simulink model "ES250A_BattVltg"  (R2013b)
settings: Solver=ode45  StartTime=0.0  StopTime=Inf  RelTol=1e-3
values from neighbouring files (symbols this model uses):
  BattVltgCorrlnSysMinVltg = DataDict.ImprtdCal    [ES250A_BattVltg_DataDict.m]
  BattVltgSwdMax = DataDict.Calibration    [ES250A_BattVltg_DataDict.m]
  BRDGFLTVLTG_VOLT_F32 = DataDict.Constant    [ES250A_BattVltg_DataDict.m]
  BrdgVltgMax = DataDict.Calibration    [ES250A_BattVltg_DataDict.m]
settings Model: Creator=NZG49T  LastModifiedBy=nzg49t

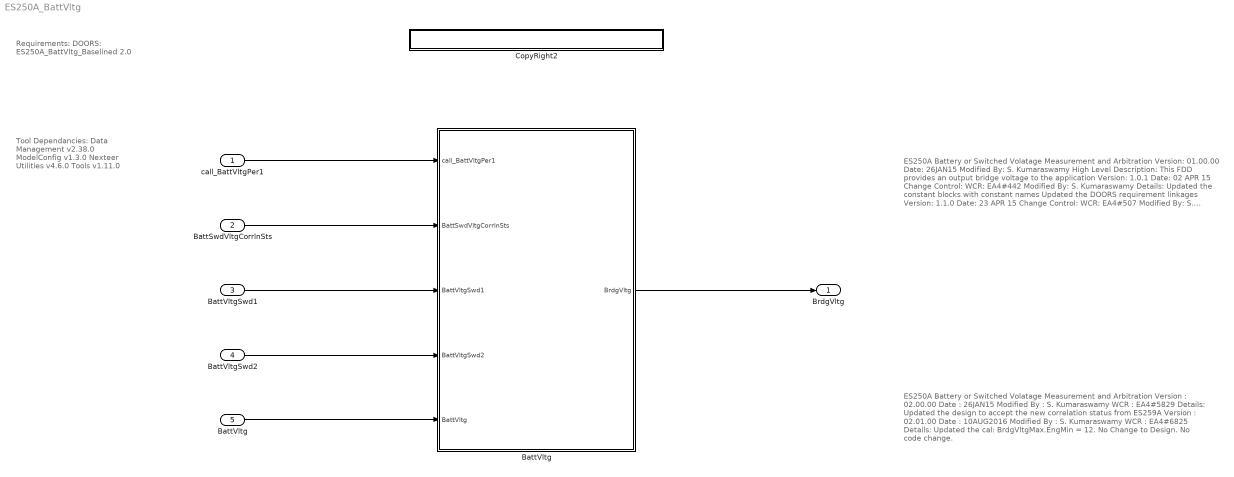
== system ES250A_BattVltg ==
  note: ES250A Battery or Switched Volatage Measurement and Arbitration
      |
      | Version: 01.00.00
      | Date: 26JAN15
      | Modified By: S. Kumaraswamy
      |
      | High Level Description:
      | This FDD provides an output bridge voltage to the application
      |
      | Version: 1.0.1
      | Date: 02 APR 15
      | Change Control: WCR: EA4#442
      | Modified By: S. Kumaraswamy
      | Details:
      | 	Updated the constant blocks with constant names
      | 	Updated the DOORS requirement linkages
      |
      | Version: 1.1.0
      | Date: 23 APR 15
      | Change Control: WCR: EA4#507
      | Modified By: S. Kumaraswamy
      | Details:
      | 	Updated the ES250A_BattVltg_DataDict.m file to change the range on inputs
  note: Tool Dependancies:
      |
      |    Data Management v2.38.0
      |    ModelConfig v1.3.0
      |    Nexteer Utilities v4.6.0
      |    Tools v1.11.0
  note: Requirements:
      |
      | DOORS: ES250A_BattVltg_Baselined 2.0
  note: ES250A Battery or Switched Volatage Measurement and Arbitration
      |
      | Version		: 02.00.00
      | Date		: 26JAN15
      | Modified By	: S. Kumaraswamy
      | WCR		: EA4#5829
      | Details:
      | 	Updated the design to accept the new correlation status from ES259A
      |
      | Version		: 02.01.00
      | Date		: 10AUG2016
      | Modified By	: S. Kumaraswamy
      | WCR		: EA4#6825
      | Details:
      | 	Updated the cal: BrdgVltgMax.EngMin = 12.
      | 	No Change to Design. No code change.
  call_BattVltgPer1 : Inport
  BattSwdVltgCorrlnSts : Inport  RequirementInfo={'linktype_rmi_doors' '000089be (/ESG Group/FDD Module Requirements/ES FDDs/ES-250A Battery and Switched Battery New Template)' '#ES250A_59' 'true' 'REQ:ES250A_59' '' } %GIDa_a11c860d_d132_4daf_a264_4400bd00e18c  Port=2
  BattVltgSwd1 : Inport  RequirementInfo={'linktype_rmi_doors' '000089be (/ESG Group/FDD Module Requirements/ES FDDs/ES-250A Battery and Switched Battery New Template)' '#ES250A_49' 'true' 'REQ:ES250A_49' '' } %GIDa_91354ed7_7d91_4356_a4ba_a513af450a0f  Port=3
  BattVltgSwd2 : Inport  RequirementInfo={'linktype_rmi_doors' '000089be (/ESG Group/FDD Module Requirements/ES FDDs/ES-250A Battery and Switched Battery New Template)' '#ES250A_60' 'true' 'REQ:ES250A_60' '' } %GIDa_49a2a00d_979f_48d9_9651_cd1224b822ec  Port=4
  "BattVltg " : Inport  RequirementInfo={'linktype_rmi_doors' '000089be (/ESG Group/FDD Module Requirements/ES FDDs/ES-250A Battery and Switched Battery New Template)' '#ES250A_48' 'true' 'REQ:ES250A_48' '' } %GIDa_3012d6f7_103b_47aa_89dd_d3628ff57ae0  Port=5
  BattVltg : Subsystem
  CopyRight2 : Subsystem  Description=|  mask(Copyright Information){none=on}
      | Copyright info block.                                               
      |                                                                     
      | Place copyright information at the top of every subsystem in design.
      mask prompts: none "No parameters"
      mask help: Place copyright information at the top of every subsystem in design.
      mask Display:
      | NxtrConf = 'Nexteer Confidential';
      | 
      | sys = bdroot; %handle for the current model ("system")
      | first = get_param(sys,'Created');
      | first = first(end-3:end);  %year is last four digits
      | 
      | last = get_param(sys,'LastModifiedDate');
      | if isempty(last)
      |     last = datestr(now,'yyyy');
      | else
      |     last = last(end-3:end);
      | end
      | 
      | if strcmp(first,last)
      |     fprintf('%s -- Copyright %s Nexteer',NxtrConf,first)
      | else
      |     fprintf('%s -- %s%s- %s Nexteer',NxtrConf,char(169),first,last)
      | end
  BrdgVltg : Outport  RequirementInfo={'linktype_rmi_doors' '000089be (/ESG Group/FDD Module Requirements/ES FDDs/ES-250A Battery and Switched Battery New Template)' '#ES250A_51' 'true' 'REQ:ES250A_51' '' } %GIDa_b80be137_a87b_4a79_92b7_89eced009269
  wires:
  BattVltg/1(BrdgVltg) -> BrdgVltg/1
  call_BattVltgPer1/1 -> BattVltg/1(call_BattVltgPer1)
  BattSwdVltgCorrlnSts/1 -> BattVltg/2(BattSwdVltgCorrlnSts)
  BattVltgSwd1/1 -> BattVltg/3(BattVltgSwd1)
  BattVltgSwd2/1 -> BattVltg/4(BattVltgSwd2)
  "BattVltg "/1 -> BattVltg/5(BattVltg)

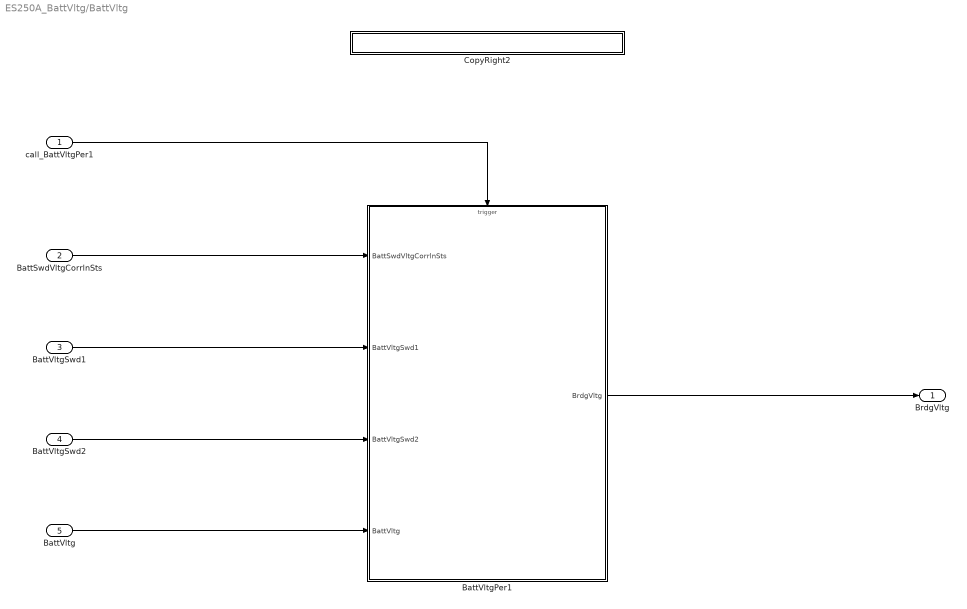
== system ES250A_BattVltg/BattVltg ==
  call_BattVltgPer1 : Inport
  BattSwdVltgCorrlnSts : Inport  RequirementInfo={'linktype_rmi_doors' '000089be (/ESG Group/FDD Module Requirements/ES FDDs/ES-250A Battery and Switched Battery New Template)' '#ES250A_59' 'true' 'REQ:ES250A_59' '' } %GIDa_e8385414_c5b7_4a96_916c_eabf55c4b14f  Port=2
  BattVltgSwd1 : Inport  RequirementInfo={'linktype_rmi_doors' '000089be (/ESG Group/FDD Module Requirements/ES FDDs/ES-250A Battery and Switched Battery New Template)' '#ES250A_49' 'true' 'REQ:ES250A_49' '' } %GIDa_5d2ad728_7230_4611_be80_0b164196a4c4  Port=3
  BattVltgSwd2 : Inport  RequirementInfo={'linktype_rmi_doors' '000089be (/ESG Group/FDD Module Requirements/ES FDDs/ES-250A Battery and Switched Battery New Template)' '#ES250A_60' 'true' 'REQ:ES250A_60' '' } %GIDa_aca025b3_6872_471e_9ce2_4632c3bd27ab  Port=4
  BattVltg : Inport  RequirementInfo={'linktype_rmi_doors' '000089be (/ESG Group/FDD Module Requirements/ES FDDs/ES-250A Battery and Switched Battery New Template)' '#ES250A_48' 'true' 'REQ:ES250A_48' '' } %GIDa_446049f3_a572_45b9_9ea0_5a0b2ee9b9f3  Port=5
  BattVltgPer1 : Subsystem
  CopyRight2 : Subsystem  Description=|  mask(Copyright Information){none=on}
      | Copyright info block.                                               
      |                                                                     
      | Place copyright information at the top of every subsystem in design.
      mask prompts: none "No parameters"
      mask help: Place copyright information at the top of every subsystem in design.
      mask Display:
      | NxtrConf = 'Nexteer Confidential';
      | 
      | sys = bdroot; %handle for the current model ("system")
      | first = get_param(sys,'Created');
      | first = first(end-3:end);  %year is last four digits
      | 
      | last = get_param(sys,'LastModifiedDate');
      | if isempty(last)
      |     last = datestr(now,'yyyy');
      | else
      |     last = last(end-3:end);
      | end
      | 
      | if strcmp(first,last)
      |     fprintf('%s -- Copyright %s Nexteer',NxtrConf,first)
      | else
      |     fprintf('%s -- %s%s- %s Nexteer',NxtrConf,char(169),first,last)
      | end
  BrdgVltg : Outport  RequirementInfo={'linktype_rmi_doors' '000089be (/ESG Group/FDD Module Requirements/ES FDDs/ES-250A Battery and Switched Battery New Template)' '#ES250A_51' 'true' 'REQ:ES250A_51' '' } %GIDa_1df96ea3_bed0_4e73_9e35_964b8173dbf2
  wires:
  call_BattVltgPer1/1 -> BattVltgPer1/Trigger
  BattVltgSwd2/1 -> BattVltgPer1/3(BattVltgSwd2)
  BattVltgSwd1/1 -> BattVltgPer1/2(BattVltgSwd1)
  BattSwdVltgCorrlnSts/1 -> BattVltgPer1/1(BattSwdVltgCorrlnSts)
  BattVltg/1 -> BattVltgPer1/4(BattVltg)
  BattVltgPer1/1(BrdgVltg) -> BrdgVltg/1

== system ES250A_BattVltg/CopyRight2 ==

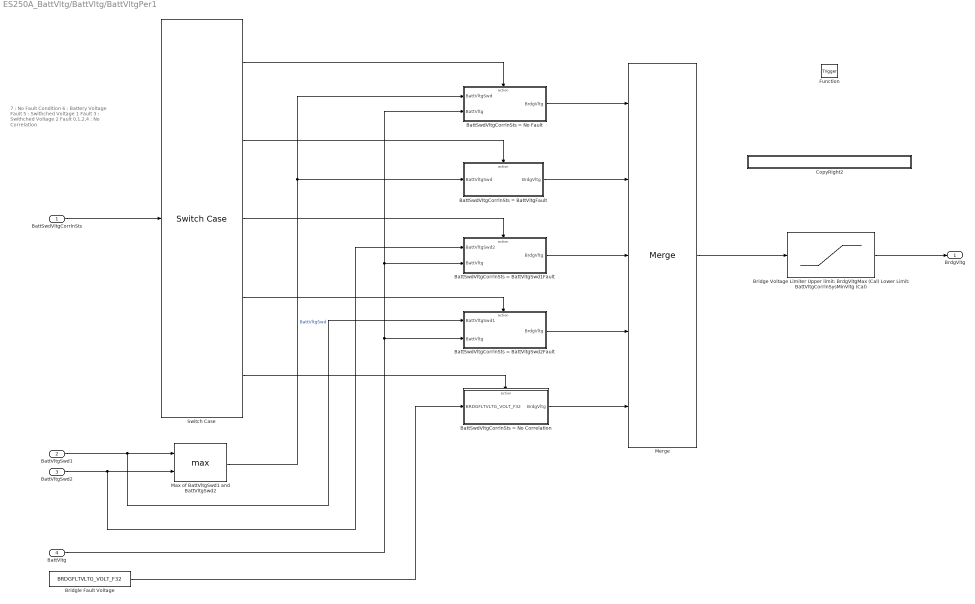
== system ES250A_BattVltg/BattVltg/BattVltgPer1 ==
  note: 7		: No Fault Condition
      | 6		: Battery Voltage Fault
      | 5		: Swithched Voltage 1 Fault
      | 3		: Swithched Voltage 2 Fault
      | 0,1,2,4	: No Correlation
  BattSwdVltgCorrlnSts : Inport
  BattVltgSwd1 : Inport  Port=2
  BattVltgSwd2 : Inport  Port=3
  BattVltg : Inport  Port=4
  Function : TriggerPort  TriggerType=function-call
  BattSwdVltgCorrlnSts = BattVltgFault : Subsystem  RequirementInfo={'linktype_rmi_doors' '000089be (/ESG Group/FDD Module Requirements/ES FDDs/ES-250A Battery and Switched Battery New Template)' '#ES250A_70' 'true' 'REQ:ES250A_70' '' } %GIDa_1e80a747_e46b_4fae_a462_c14971ea2063  TreatAsAtomicUnit=on
  BattSwdVltgCorrlnSts = BattVltgSwd1Fault : Subsystem  RequirementInfo={'linktype_rmi_doors' '000089be (/E-STEER Core/SubSystem Specifications/Electrical Actuator/Control Module/FDD Module Requirements/EA4/ES250A_BattVltg)' '#ES250A_71' 'true' 'REQ:ES250A_71' '' ; 'linktype_rmi_doors' '000089be (/E-STEER Core/SubSystem Specifications/Electrical Actuator/Control Module/FDD Module Requirements/EA4/ES250A_BattVltg)' '#ES250A_74' 'true' 'REQ:ES250A_74' '' } %GIDa_d2edab66_9a38_4fa0_805c_5347de679304  TreatAsAtomicUnit=on
  BattSwdVltgCorrlnSts = BattVltgSwd2Fault : Subsystem  RequirementInfo={'linktype_rmi_doors' '000089be (/E-STEER Core/SubSystem Specifications/Electrical Actuator/Control Module/FDD Module Requirements/EA4/ES250A_BattVltg)' '#ES250A_71' 'true' 'REQ:ES250A_71' '' ; 'linktype_rmi_doors' '000089be (/E-STEER Core/SubSystem Specifications/Electrical Actuator/Control Module/FDD Module Requirements/EA4/ES250A_BattVltg)' '#ES250A_73' 'true' 'REQ:ES250A_73' '' } %GIDa_b90dafad_55ba_4f29_80ae_7ffeed94569b  TreatAsAtomicUnit=on
  BattSwdVltgCorrlnSts = No Correlation : Subsystem  RequirementInfo={'linktype_rmi_doors' '000089be (/E-STEER Core/SubSystem Specifications/Electrical Actuator/Control Module/FDD Module Requirements/EA4/ES250A_BattVltg)' '#ES250A_69' 'true' 'REQ:ES250A_69' '' } %GIDa_00f660ee_d345_4718_bc3f_0f212dfcf13e  TreatAsAtomicUnit=on
  BattSwdVltgCorrlnSts = No Fault : Subsystem  RequirementInfo={'linktype_rmi_doors' '000089be (/E-STEER Core/SubSystem Specifications/Electrical Actuator/Control Module/FDD Module Requirements/EA4/ES250A_BattVltg)' '#ES250A_71' 'true' 'REQ:ES250A_71' '' ; 'linktype_rmi_doors' '000089be (/E-STEER Core/SubSystem Specifications/Electrical Actuator/Control Module/FDD Module Requirements/EA4/ES250A_BattVltg)' '#ES250A_72' 'true' 'REQ:ES250A_72' '' } %GIDa_5403e315_0859_46da_b9ef_39481c3f6656  TreatAsAtomicUnit=on
  Bridge Voltage Limiter Upper limit: BrdgVltgMax (Cal) Lower Limit: BattVltgCorrlnSysMinVltg (Cal) : Saturate  RequirementInfo={'linktype_rmi_doors' '000089be (/ESG Group/FDD Module Requirements/ES FDDs/ES-250A Battery and Switched Battery New Template)' '#ES250A_77' 'true' 'REQ:ES250A_77' '' } %GIDa_140e9a93_79da_47f9_8f89_a5c416ccae8e  UpperLimit=BrdgVltgMax  LowerLimit=BattVltgCorrlnSysMinVltg
  Bridgle Fault Voltage : Constant  Value=BRDGFLTVLTG_VOLT_F32  OutDataTypeStr=single
  CopyRight2 : Subsystem  Description=|  mask(Copyright Information){none=on}
      | Copyright info block.                                               
      |                                                                     
      | Place copyright information at the top of every subsystem in design.
      mask prompts: none "No parameters"
      mask help: Place copyright information at the top of every subsystem in design.
      mask Display:
      | NxtrConf = 'Nexteer Confidential';
      | 
      | sys = bdroot; %handle for the current model ("system")
      | first = get_param(sys,'Created');
      | first = first(end-3:end);  %year is last four digits
      | 
      | last = get_param(sys,'LastModifiedDate');
      | if isempty(last)
      |     last = datestr(now,'yyyy');
      | else
      |     last = last(end-3:end);
      | end
      | 
      | if strcmp(first,last)
      |     fprintf('%s -- Copyright %s Nexteer',NxtrConf,first)
      | else
      |     fprintf('%s -- %s%s- %s Nexteer',NxtrConf,char(169),first,last)
      | end
  Max of BattVltgSwd1 and BattVltgSwd2 : MinMax  Function=max  Inputs=2  ZeroCross=off
  Merge : Merge  Inputs=5
  Switch Case : SwitchCase  CaseConditions={7,6,5,3}
  BrdgVltg : Outport
  wires:
  BattSwdVltgCorrlnSts/1 -> Switch Case/1
  BattVltgSwd1/1 -> BattSwdVltgCorrlnSts = BattVltgSwd2Fault/1(BattVltgSwd1), Max of BattVltgSwd1 and BattVltgSwd2/1
  Max of BattVltgSwd1 and BattVltgSwd2/1 -> BattSwdVltgCorrlnSts = No Fault/1(BattVltgSwd), BattSwdVltgCorrlnSts = BattVltgFault/1(BattVltgSwd)  "BattVltgSwd"
  Switch Case/5 -> BattSwdVltgCorrlnSts = No Correlation/Action
  BattVltgSwd2/1 -> Max of BattVltgSwd1 and BattVltgSwd2/2, BattSwdVltgCorrlnSts = BattVltgSwd1Fault/1(BattVltgSwd2)
  BattSwdVltgCorrlnSts = No Correlation/1(BrdgVltg) -> Merge/5
  Bridgle Fault Voltage/1 -> BattSwdVltgCorrlnSts = No Correlation/1(BRDGFLTVLTG_VOLT_F32)
  BattVltg/1 -> BattSwdVltgCorrlnSts = No Fault/2(BattVltg), BattSwdVltgCorrlnSts = BattVltgSwd1Fault/2(BattVltg), BattSwdVltgCorrlnSts = BattVltgSwd2Fault/2(BattVltg)
  BattSwdVltgCorrlnSts = No Fault/1(BrdgVltg) -> Merge/1
  Switch Case/1 -> BattSwdVltgCorrlnSts = No Fault/Action
  Merge/1 -> Bridge Voltage Limiter Upper limit: BrdgVltgMax (Cal) Lower Limit: BattVltgCorrlnSysMinVltg (Cal)/1
  Bridge Voltage Limiter Upper limit: BrdgVltgMax (Cal) Lower Limit: BattVltgCorrlnSysMinVltg (Cal)/1 -> BrdgVltg/1
  Switch Case/2 -> BattSwdVltgCorrlnSts = BattVltgFault/Action
  Switch Case/3 -> BattSwdVltgCorrlnSts = BattVltgSwd1Fault/Action
  Switch Case/4 -> BattSwdVltgCorrlnSts = BattVltgSwd2Fault/Action
  BattSwdVltgCorrlnSts = BattVltgFault/1(BrdgVltg) -> Merge/2
  BattSwdVltgCorrlnSts = BattVltgSwd1Fault/1(BrdgVltg) -> Merge/3
  BattSwdVltgCorrlnSts = BattVltgSwd2Fault/1(BrdgVltg) -> Merge/4

== system ES250A_BattVltg/BattVltg/CopyRight2 ==

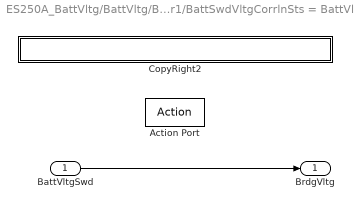
== system ES250A_BattVltg/BattVltg/BattVltgPer1/BattSwdVltgCorrlnSts = BattVltgFault ==
  BattVltgSwd : Inport
  Action Port : ActionPort  ActionType=case
  CopyRight2 : Subsystem  Description=|  mask(Copyright Information){none=on}
      | Copyright info block.                                               
      |                                                                     
      | Place copyright information at the top of every subsystem in design.
      mask prompts: none "No parameters"
      mask help: Place copyright information at the top of every subsystem in design.
      mask Display:
      | NxtrConf = 'Nexteer Confidential';
      | 
      | sys = bdroot; %handle for the current model ("system")
      | first = get_param(sys,'Created');
      | first = first(end-3:end);  %year is last four digits
      | 
      | last = get_param(sys,'LastModifiedDate');
      | if isempty(last)
      |     last = datestr(now,'yyyy');
      | else
      |     last = last(end-3:end);
      | end
      | 
      | if strcmp(first,last)
      |     fprintf('%s -- Copyright %s Nexteer',NxtrConf,first)
      | else
      |     fprintf('%s -- %s%s- %s Nexteer',NxtrConf,char(169),first,last)
      | end
  BrdgVltg : Outport
  wires:
  BattVltgSwd/1 -> BrdgVltg/1

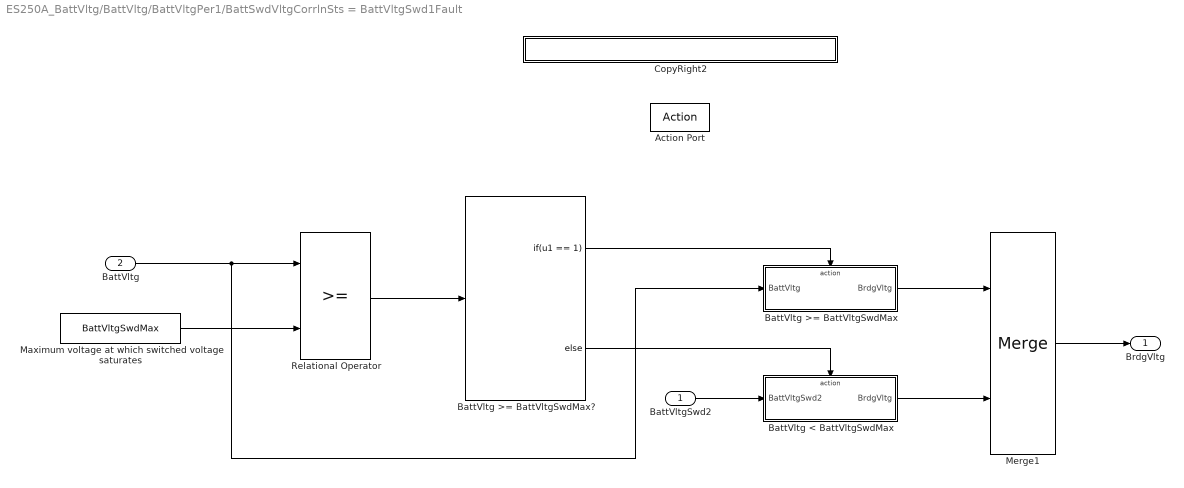
== system ES250A_BattVltg/BattVltg/BattVltgPer1/BattSwdVltgCorrlnSts = BattVltgSwd1Fault ==
  BattVltgSwd2 : Inport
  BattVltg : Inport  Port=2
  Action Port : ActionPort  ActionType=case
  BattVltg < BattVltgSwdMax : Subsystem  RequirementInfo={'linktype_rmi_doors' '000089be (/ESG Group/FDD Module Requirements/ES FDDs/ES-250A Battery and Switched Battery New Template)' '#ES250A_74' 'true' 'REQ:ES250A_74' '' } %GIDa_07292b91_eb89_4c3a_b17b_a04f2de4c9d3  TreatAsAtomicUnit=on
  BattVltg >= BattVltgSwdMax : Subsystem  RequirementInfo={'linktype_rmi_doors' '000089be (/ESG Group/FDD Module Requirements/ES FDDs/ES-250A Battery and Switched Battery New Template)' '#ES250A_71' 'true' 'REQ:ES250A_71' '' } %GIDa_bcfe97d8_f970_4b6a_b766_e1f79e97ff7b  TreatAsAtomicUnit=on
  BattVltg >= BattVltgSwdMax? : If  IfExpression=u1 == 1
  CopyRight2 : Subsystem  Description=|  mask(Copyright Information){none=on}
      | Copyright info block.                                               
      |                                                                     
      | Place copyright information at the top of every subsystem in design.
      mask prompts: none "No parameters"
      mask help: Place copyright information at the top of every subsystem in design.
      mask Display:
      | NxtrConf = 'Nexteer Confidential';
      | 
      | sys = bdroot; %handle for the current model ("system")
      | first = get_param(sys,'Created');
      | first = first(end-3:end);  %year is last four digits
      | 
      | last = get_param(sys,'LastModifiedDate');
      | if isempty(last)
      |     last = datestr(now,'yyyy');
      | else
      |     last = last(end-3:end);
      | end
      | 
      | if strcmp(first,last)
      |     fprintf('%s -- Copyright %s Nexteer',NxtrConf,first)
      | else
      |     fprintf('%s -- %s%s- %s Nexteer',NxtrConf,char(169),first,last)
      | end
  Maximum voltage at which switched voltage saturates : Constant  Value=BattVltgSwdMax  OutDataTypeStr=single
  Merge1 : Merge
  Relational Operator : RelationalOperator  OutDataTypeStr=boolean
  BrdgVltg : Outport
  wires:
  BattVltg >= BattVltgSwdMax?/1 -> BattVltg >= BattVltgSwdMax/Action
  BattVltg >= BattVltgSwdMax?/2 -> BattVltg < BattVltgSwdMax/Action
  BattVltgSwd2/1 -> BattVltg < BattVltgSwdMax/1(BattVltgSwd2)
  BattVltg >= BattVltgSwdMax/1(BrdgVltg) -> Merge1/1
  BattVltg < BattVltgSwdMax/1(BrdgVltg) -> Merge1/2
  Merge1/1 -> BrdgVltg/1
  BattVltg/1 -> BattVltg >= BattVltgSwdMax/1(BattVltg), Relational Operator/1
  Maximum voltage at which switched voltage saturates/1 -> Relational Operator/2
  Relational Operator/1 -> BattVltg >= BattVltgSwdMax?/1

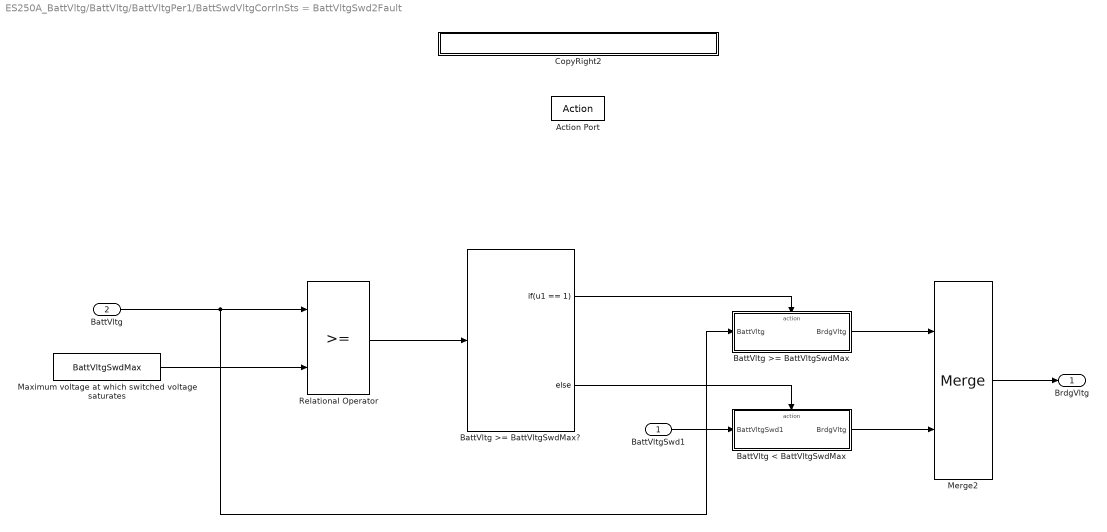
== system ES250A_BattVltg/BattVltg/BattVltgPer1/BattSwdVltgCorrlnSts = BattVltgSwd2Fault ==
  BattVltgSwd1 : Inport
  BattVltg : Inport  Port=2
  Action Port : ActionPort  ActionType=case
  BattVltg < BattVltgSwdMax : Subsystem  RequirementInfo={'linktype_rmi_doors' '000089be (/ESG Group/FDD Module Requirements/ES FDDs/ES-250A Battery and Switched Battery New Template)' '#ES250A_73' 'true' 'REQ:ES250A_73' '' } %GIDa_307ba01f_b79a_432e_bfbc_716903f8ff55  TreatAsAtomicUnit=on
  BattVltg >= BattVltgSwdMax : Subsystem  RequirementInfo={'linktype_rmi_doors' '000089be (/ESG Group/FDD Module Requirements/ES FDDs/ES-250A Battery and Switched Battery New Template)' '#ES250A_71' 'true' 'REQ:ES250A_71' '' } %GIDa_ba8018fa_2f9e_46d8_a7b7_d203f8c6e12a  TreatAsAtomicUnit=on
  BattVltg >= BattVltgSwdMax? : If  IfExpression=u1 == 1
  CopyRight2 : Subsystem  Description=|  mask(Copyright Information){none=on}
      | Copyright info block.                                               
      |                                                                     
      | Place copyright information at the top of every subsystem in design.
      mask prompts: none "No parameters"
      mask help: Place copyright information at the top of every subsystem in design.
      mask Display:
      | NxtrConf = 'Nexteer Confidential';
      | 
      | sys = bdroot; %handle for the current model ("system")
      | first = get_param(sys,'Created');
      | first = first(end-3:end);  %year is last four digits
      | 
      | last = get_param(sys,'LastModifiedDate');
      | if isempty(last)
      |     last = datestr(now,'yyyy');
      | else
      |     last = last(end-3:end);
      | end
      | 
      | if strcmp(first,last)
      |     fprintf('%s -- Copyright %s Nexteer',NxtrConf,first)
      | else
      |     fprintf('%s -- %s%s- %s Nexteer',NxtrConf,char(169),first,last)
      | end
  Maximum voltage at which switched voltage saturates : Constant  Value=BattVltgSwdMax  OutDataTypeStr=single
  Merge2 : Merge
  Relational Operator : RelationalOperator  OutDataTypeStr=boolean
  BrdgVltg : Outport
  wires:
  BattVltg/1 -> BattVltg >= BattVltgSwdMax/1(BattVltg), Relational Operator/1
  BattVltg >= BattVltgSwdMax?/1 -> BattVltg >= BattVltgSwdMax/Action
  BattVltg >= BattVltgSwdMax?/2 -> BattVltg < BattVltgSwdMax/Action
  BattVltgSwd1/1 -> BattVltg < BattVltgSwdMax/1(BattVltgSwd1)
  BattVltg >= BattVltgSwdMax/1(BrdgVltg) -> Merge2/1
  BattVltg < BattVltgSwdMax/1(BrdgVltg) -> Merge2/2
  Merge2/1 -> BrdgVltg/1
  Maximum voltage at which switched voltage saturates/1 -> Relational Operator/2
  Relational Operator/1 -> BattVltg >= BattVltgSwdMax?/1

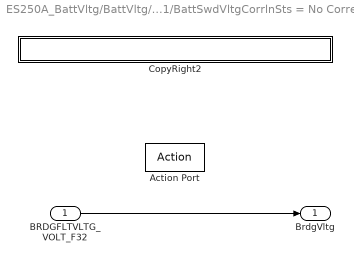
== system ES250A_BattVltg/BattVltg/BattVltgPer1/BattSwdVltgCorrlnSts = No Correlation ==
  BRDGFLTVLTG_VOLT_F32 : Inport
  Action Port : ActionPort  ActionType=default
  CopyRight2 : Subsystem  Description=|  mask(Copyright Information){none=on}
      | Copyright info block.                                               
      |                                                                     
      | Place copyright information at the top of every subsystem in design.
      mask prompts: none "No parameters"
      mask help: Place copyright information at the top of every subsystem in design.
      mask Display:
      | NxtrConf = 'Nexteer Confidential';
      | 
      | sys = bdroot; %handle for the current model ("system")
      | first = get_param(sys,'Created');
      | first = first(end-3:end);  %year is last four digits
      | 
      | last = get_param(sys,'LastModifiedDate');
      | if isempty(last)
      |     last = datestr(now,'yyyy');
      | else
      |     last = last(end-3:end);
      | end
      | 
      | if strcmp(first,last)
      |     fprintf('%s -- Copyright %s Nexteer',NxtrConf,first)
      | else
      |     fprintf('%s -- %s%s- %s Nexteer',NxtrConf,char(169),first,last)
      | end
  BrdgVltg : Outport
  wires:
  BRDGFLTVLTG_VOLT_F32/1 -> BrdgVltg/1

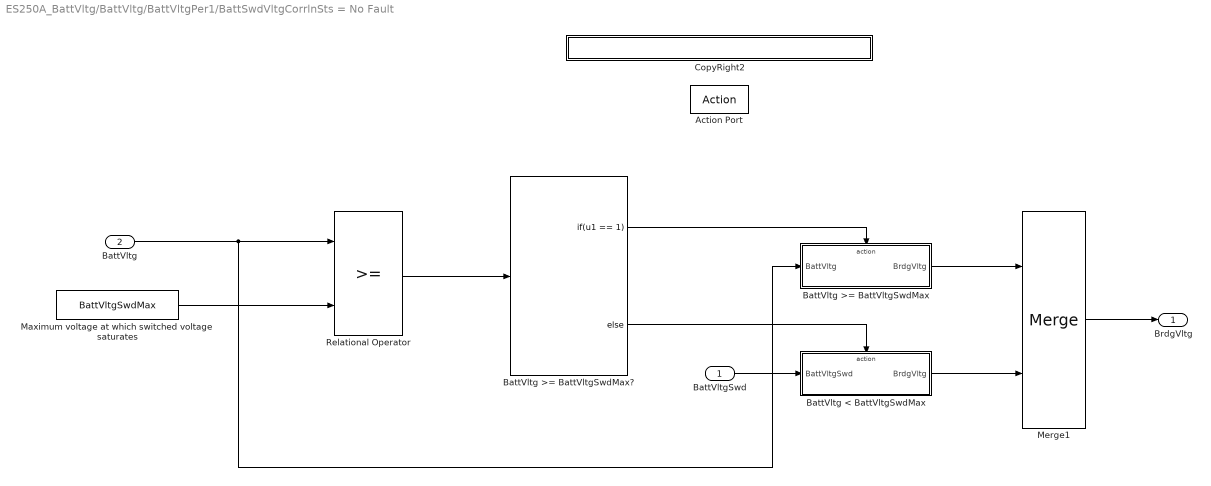
== system ES250A_BattVltg/BattVltg/BattVltgPer1/BattSwdVltgCorrlnSts = No Fault ==
  BattVltgSwd : Inport
  BattVltg : Inport  Port=2
  Action Port : ActionPort  ActionType=case
  BattVltg < BattVltgSwdMax : Subsystem  RequirementInfo={'linktype_rmi_doors' '000089be (/ESG Group/FDD Module Requirements/ES FDDs/ES-250A Battery and Switched Battery New Template)' '#ES250A_72' 'true' 'REQ:ES250A_72' '' } %GIDa_fc36a75c_2fdb_43c4_a531_122c5df0c909  TreatAsAtomicUnit=on
  BattVltg >= BattVltgSwdMax : Subsystem  RequirementInfo={'linktype_rmi_doors' '000089be (/ESG Group/FDD Module Requirements/ES FDDs/ES-250A Battery and Switched Battery New Template)' '#ES250A_71' 'true' 'REQ:ES250A_71' '' } %GIDa_4f6ba4fb_a439_4a78_8be4_0d81f695ed1e  TreatAsAtomicUnit=on
  BattVltg >= BattVltgSwdMax? : If  IfExpression=u1 == 1
  CopyRight2 : Subsystem  Description=|  mask(Copyright Information){none=on}
      | Copyright info block.                                               
      |                                                                     
      | Place copyright information at the top of every subsystem in design.
      mask prompts: none "No parameters"
      mask help: Place copyright information at the top of every subsystem in design.
      mask Display:
      | NxtrConf = 'Nexteer Confidential';
      | 
      | sys = bdroot; %handle for the current model ("system")
      | first = get_param(sys,'Created');
      | first = first(end-3:end);  %year is last four digits
      | 
      | last = get_param(sys,'LastModifiedDate');
      | if isempty(last)
      |     last = datestr(now,'yyyy');
      | else
      |     last = last(end-3:end);
      | end
      | 
      | if strcmp(first,last)
      |     fprintf('%s -- Copyright %s Nexteer',NxtrConf,first)
      | else
      |     fprintf('%s -- %s%s- %s Nexteer',NxtrConf,char(169),first,last)
      | end
  Maximum voltage at which switched voltage saturates : Constant  Value=BattVltgSwdMax  OutDataTypeStr=single
  Merge1 : Merge
  Relational Operator : RelationalOperator  OutDataTypeStr=boolean
  BrdgVltg : Outport
  wires:
  BattVltg/1 -> BattVltg >= BattVltgSwdMax/1(BattVltg), Relational Operator/1
  BattVltg >= BattVltgSwdMax?/1 -> BattVltg >= BattVltgSwdMax/Action
  BattVltg >= BattVltgSwdMax?/2 -> BattVltg < BattVltgSwdMax/Action
  BattVltgSwd/1 -> BattVltg < BattVltgSwdMax/1(BattVltgSwd)
  BattVltg >= BattVltgSwdMax/1(BrdgVltg) -> Merge1/1
  BattVltg < BattVltgSwdMax/1(BrdgVltg) -> Merge1/2
  Merge1/1 -> BrdgVltg/1
  Maximum voltage at which switched voltage saturates/1 -> Relational Operator/2
  Relational Operator/1 -> BattVltg >= BattVltgSwdMax?/1

== system ES250A_BattVltg/BattVltg/BattVltgPer1/CopyRight2 ==

== system ES250A_BattVltg/BattVltg/BattVltgPer1/BattSwdVltgCorrlnSts = BattVltgFault/CopyRight2 ==

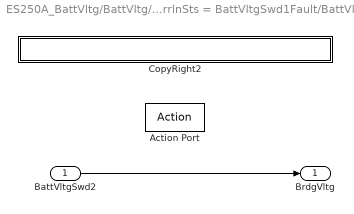
== system ES250A_BattVltg/BattVltg/BattVltgPer1/BattSwdVltgCorrlnSts = BattVltgSwd1Fault/BattVltg < BattVltgSwdMax ==
  BattVltgSwd2 : Inport
  Action Port : ActionPort  ActionType=else
  CopyRight2 : Subsystem  Description=|  mask(Copyright Information){none=on}
      | Copyright info block.                                               
      |                                                                     
      | Place copyright information at the top of every subsystem in design.
      mask prompts: none "No parameters"
      mask help: Place copyright information at the top of every subsystem in design.
      mask Display:
      | NxtrConf = 'Nexteer Confidential';
      | 
      | sys = bdroot; %handle for the current model ("system")
      | first = get_param(sys,'Created');
      | first = first(end-3:end);  %year is last four digits
      | 
      | last = get_param(sys,'LastModifiedDate');
      | if isempty(last)
      |     last = datestr(now,'yyyy');
      | else
      |     last = last(end-3:end);
      | end
      | 
      | if strcmp(first,last)
      |     fprintf('%s -- Copyright %s Nexteer',NxtrConf,first)
      | else
      |     fprintf('%s -- %s%s- %s Nexteer',NxtrConf,char(169),first,last)
      | end
  BrdgVltg : Outport
  wires:
  BattVltgSwd2/1 -> BrdgVltg/1

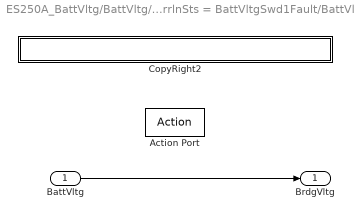
== system ES250A_BattVltg/BattVltg/BattVltgPer1/BattSwdVltgCorrlnSts = BattVltgSwd1Fault/BattVltg >= BattVltgSwdMax ==
  BattVltg : Inport
  Action Port : ActionPort  ActionType=then
  CopyRight2 : Subsystem  Description=|  mask(Copyright Information){none=on}
      | Copyright info block.                                               
      |                                                                     
      | Place copyright information at the top of every subsystem in design.
      mask prompts: none "No parameters"
      mask help: Place copyright information at the top of every subsystem in design.
      mask Display:
      | NxtrConf = 'Nexteer Confidential';
      | 
      | sys = bdroot; %handle for the current model ("system")
      | first = get_param(sys,'Created');
      | first = first(end-3:end);  %year is last four digits
      | 
      | last = get_param(sys,'LastModifiedDate');
      | if isempty(last)
      |     last = datestr(now,'yyyy');
      | else
      |     last = last(end-3:end);
      | end
      | 
      | if strcmp(first,last)
      |     fprintf('%s -- Copyright %s Nexteer',NxtrConf,first)
      | else
      |     fprintf('%s -- %s%s- %s Nexteer',NxtrConf,char(169),first,last)
      | end
  BrdgVltg : Outport
  wires:
  BattVltg/1 -> BrdgVltg/1

== system ES250A_BattVltg/BattVltg/BattVltgPer1/BattSwdVltgCorrlnSts = BattVltgSwd1Fault/CopyRight2 ==

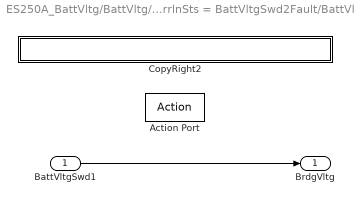
== system ES250A_BattVltg/BattVltg/BattVltgPer1/BattSwdVltgCorrlnSts = BattVltgSwd2Fault/BattVltg < BattVltgSwdMax ==
  BattVltgSwd1 : Inport
  Action Port : ActionPort  ActionType=else
  CopyRight2 : Subsystem  Description=|  mask(Copyright Information){none=on}
      | Copyright info block.                                               
      |                                                                     
      | Place copyright information at the top of every subsystem in design.
      mask prompts: none "No parameters"
      mask help: Place copyright information at the top of every subsystem in design.
      mask Display:
      | NxtrConf = 'Nexteer Confidential';
      | 
      | sys = bdroot; %handle for the current model ("system")
      | first = get_param(sys,'Created');
      | first = first(end-3:end);  %year is last four digits
      | 
      | last = get_param(sys,'LastModifiedDate');
      | if isempty(last)
      |     last = datestr(now,'yyyy');
      | else
      |     last = last(end-3:end);
      | end
      | 
      | if strcmp(first,last)
      |     fprintf('%s -- Copyright %s Nexteer',NxtrConf,first)
      | else
      |     fprintf('%s -- %s%s- %s Nexteer',NxtrConf,char(169),first,last)
      | end
  BrdgVltg : Outport
  wires:
  BattVltgSwd1/1 -> BrdgVltg/1

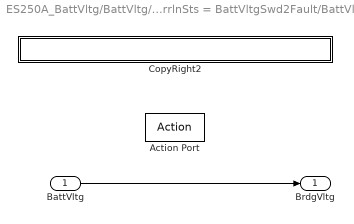
== system ES250A_BattVltg/BattVltg/BattVltgPer1/BattSwdVltgCorrlnSts = BattVltgSwd2Fault/BattVltg >= BattVltgSwdMax ==
  BattVltg : Inport
  Action Port : ActionPort  ActionType=then
  CopyRight2 : Subsystem  Description=|  mask(Copyright Information){none=on}
      | Copyright info block.                                               
      |                                                                     
      | Place copyright information at the top of every subsystem in design.
      mask prompts: none "No parameters"
      mask help: Place copyright information at the top of every subsystem in design.
      mask Display:
      | NxtrConf = 'Nexteer Confidential';
      | 
      | sys = bdroot; %handle for the current model ("system")
      | first = get_param(sys,'Created');
      | first = first(end-3:end);  %year is last four digits
      | 
      | last = get_param(sys,'LastModifiedDate');
      | if isempty(last)
      |     last = datestr(now,'yyyy');
      | else
      |     last = last(end-3:end);
      | end
      | 
      | if strcmp(first,last)
      |     fprintf('%s -- Copyright %s Nexteer',NxtrConf,first)
      | else
      |     fprintf('%s -- %s%s- %s Nexteer',NxtrConf,char(169),first,last)
      | end
  BrdgVltg : Outport
  wires:
  BattVltg/1 -> BrdgVltg/1

== system ES250A_BattVltg/BattVltg/BattVltgPer1/BattSwdVltgCorrlnSts = BattVltgSwd2Fault/CopyRight2 ==

== system ES250A_BattVltg/BattVltg/BattVltgPer1/BattSwdVltgCorrlnSts = No Correlation/CopyRight2 ==

== system ES250A_BattVltg/BattVltg/BattVltgPer1/BattSwdVltgCorrlnSts = No Fault/BattVltg < BattVltgSwdMax ==
  BattVltgSwd : Inport
  Action Port : ActionPort  ActionType=else
  CopyRight2 : Subsystem  Description=|  mask(Copyright Information){none=on}
      | Copyright info block.                                               
      |                                                                     
      | Place copyright information at the top of every subsystem in design.
      mask prompts: none "No parameters"
      mask help: Place copyright information at the top of every subsystem in design.
      mask Display:
      | NxtrConf = 'Nexteer Confidential';
      | 
      | sys = bdroot; %handle for the current model ("system")
      | first = get_param(sys,'Created');
      | first = first(end-3:end);  %year is last four digits
      | 
      | last = get_param(sys,'LastModifiedDate');
      | if isempty(last)
      |     last = datestr(now,'yyyy');
      | else
      |     last = last(end-3:end);
      | end
      | 
      | if strcmp(first,last)
      |     fprintf('%s -- Copyright %s Nexteer',NxtrConf,first)
      | else
      |     fprintf('%s -- %s%s- %s Nexteer',NxtrConf,char(169),first,last)
      | end
  BrdgVltg : Outport
  wires:
  BattVltgSwd/1 -> BrdgVltg/1

== system ES250A_BattVltg/BattVltg/BattVltgPer1/BattSwdVltgCorrlnSts = No Fault/BattVltg >= BattVltgSwdMax ==
  BattVltg : Inport
  Action Port : ActionPort  ActionType=then
  CopyRight2 : Subsystem  Description=|  mask(Copyright Information){none=on}
      | Copyright info block.                                               
      |                                                                     
      | Place copyright information at the top of every subsystem in design.
      mask prompts: none "No parameters"
      mask help: Place copyright information at the top of every subsystem in design.
      mask Display:
      | NxtrConf = 'Nexteer Confidential';
      | 
      | sys = bdroot; %handle for the current model ("system")
      | first = get_param(sys,'Created');
      | first = first(end-3:end);  %year is last four digits
      | 
      | last = get_param(sys,'LastModifiedDate');
      | if isempty(last)
      |     last = datestr(now,'yyyy');
      | else
      |     last = last(end-3:end);
      | end
      | 
      | if strcmp(first,last)
      |     fprintf('%s -- Copyright %s Nexteer',NxtrConf,first)
      | else
      |     fprintf('%s -- %s%s- %s Nexteer',NxtrConf,char(169),first,last)
      | end
  BrdgVltg : Outport
  wires:
  BattVltg/1 -> BrdgVltg/1

== system ES250A_BattVltg/BattVltg/BattVltgPer1/BattSwdVltgCorrlnSts = No Fault/CopyRight2 ==

== system ES250A_BattVltg/BattVltg/BattVltgPer1/BattSwdVltgCorrlnSts = BattVltgSwd1Fault/BattVltg < BattVltgSwdMax/CopyRight2 ==

== system ES250A_BattVltg/BattVltg/BattVltgPer1/BattSwdVltgCorrlnSts = BattVltgSwd1Fault/BattVltg >= BattVltgSwdMax/CopyRight2 ==

== system ES250A_BattVltg/BattVltg/BattVltgPer1/BattSwdVltgCorrlnSts = BattVltgSwd2Fault/BattVltg < BattVltgSwdMax/CopyRight2 ==

== system ES250A_BattVltg/BattVltg/BattVltgPer1/BattSwdVltgCorrlnSts = BattVltgSwd2Fault/BattVltg >= BattVltgSwdMax/CopyRight2 ==

== system ES250A_BattVltg/BattVltg/BattVltgPer1/BattSwdVltgCorrlnSts = No Fault/BattVltg < BattVltgSwdMax/CopyRight2 ==

== system ES250A_BattVltg/BattVltg/BattVltgPer1/BattSwdVltgCorrlnSts = No Fault/BattVltg >= BattVltgSwdMax/CopyRight2 ==
